simulink model "Digitaltwin_model"  (R2024b)
settings: Solver=ode45  StartTime=0.0  StopTime=10.0  RelTol=1e-3

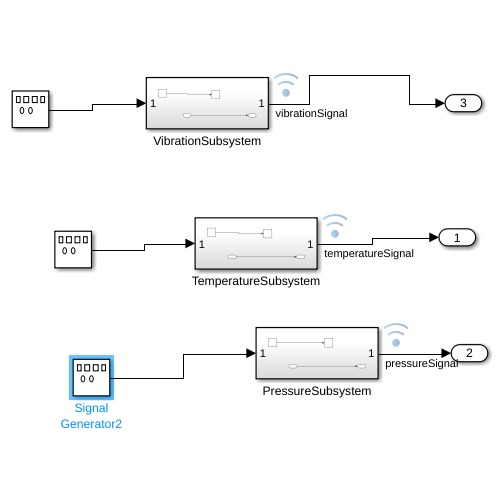
[thumbnail: Simulink's stored preview of the top-level diagram]
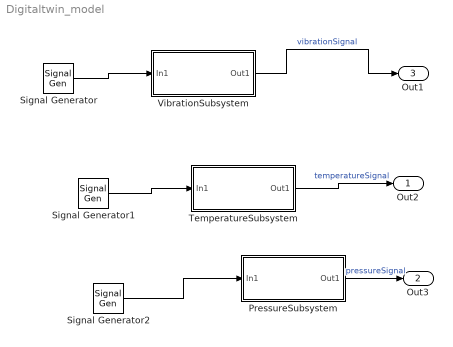
== system Digitaltwin_model ==
  PressureSubsystem : Subsystem
  Signal Generator : SignalGenerator  Units=rad/sec
  Signal Generator1 : SignalGenerator  WaveForm=sawtooth  Amplitude=3  Units=rad/sec
  Signal Generator2 : SignalGenerator  WaveForm=random  Amplitude=2  Units=rad/sec
  TemperatureSubsystem : Subsystem
  VibrationSubsystem : Subsystem
  Out2 : Outport
  Out3 : Outport  Port=2
  Out1 : Outport  Port=3
  wires:
  TemperatureSubsystem/1(Out1) -> Out2/1  "temperatureSignal"
  PressureSubsystem/1(Out1) -> Out3/1  "pressureSignal"
  VibrationSubsystem/1(Out1) -> Out1/1  "vibrationSignal"
  Signal Generator/1 -> VibrationSubsystem/1(In1)
  Signal Generator1/1 -> TemperatureSubsystem/1(In1)
  Signal Generator2/1 -> PressureSubsystem/1(In1)

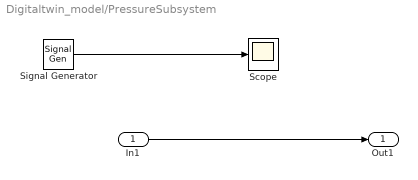
== system Digitaltwin_model/PressureSubsystem ==
  In1 : Inport
  Scope : Scope
  Signal Generator : SignalGenerator  Amplitude=5  Units=rad/sec
  Out1 : Outport
  wires:
  In1/1 -> Out1/1
  Signal Generator/1 -> Scope/1

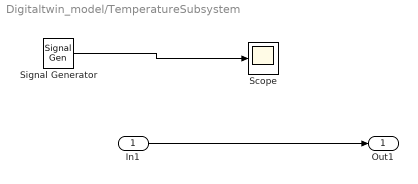
== system Digitaltwin_model/TemperatureSubsystem ==
  In1 : Inport
  Scope : Scope
  Signal Generator : SignalGenerator  Amplitude=4  Units=rad/sec
  Out1 : Outport
  wires:
  In1/1 -> Out1/1
  Signal Generator/1 -> Scope/1

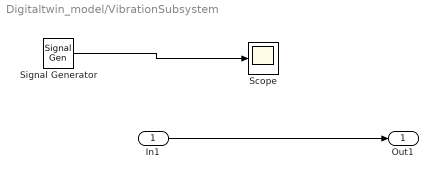
== system Digitaltwin_model/VibrationSubsystem ==
  In1 : Inport
  Scope : Scope
  Signal Generator : SignalGenerator  Amplitude=3  Units=rad/sec
  Out1 : Outport
  wires:
  Signal Generator/1 -> Scope/1
  In1/1 -> Out1/1
